simulink model "plane_stablizer_1"  (R2020b)
settings: Solver=VariableStepAuto  StartTime=0.0  StopTime=10.0  RelTol=1e-3
undefined symbols (not defined in the file): DiscIntNeverNeededParam
libraries: arduinolib x3, svdutilitieslib x1, arduinosensorlib x1
settings Model: Creator=Chas  LastModifiedBy=Chas

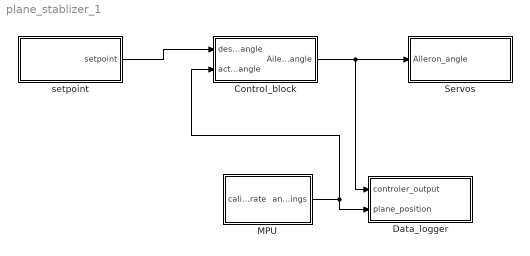
== system plane_stablizer_1 ==
  Control_block : Subsystem
  Data_logger : Subsystem
  MPU : Subsystem
  Servos : Subsystem
  setpoint : Subsystem
  wires:
  setpoint/1(setpoint) -> Control_block/1(desired_plane_angle)
  Control_block/1(Aileron_angle) -> Data_logger/1(controler_output), Servos/1(Aileron_angle)
  MPU/1(angle_of_wings) -> Control_block/2(actual_plan_angle), Data_logger/2(plane_position)

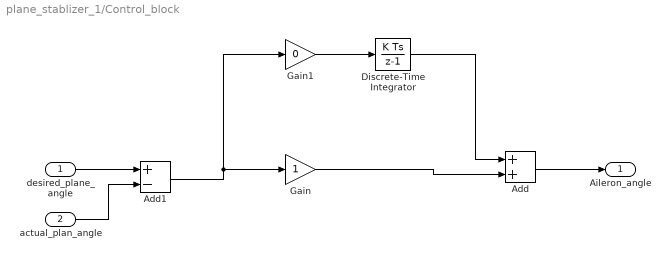
== system plane_stablizer_1/Control_block ==
  desired_plane_angle : Inport
  actual_plan_angle : Inport  Port=2
  Add : Sum
  Add1 : Sum  Inputs=+-
  Discrete-Time Integrator : DiscreteIntegrator  SampleTime=-1  ICPrevOutput=DiscIntNeverNeededParam  ICPrevScaledInput=DiscIntNeverNeededParam
  Gain : Gain
  Gain1 : Gain  Gain=0
  Aileron_angle : Outport
  wires:
  Gain1/1 -> Discrete-Time Integrator/1
  Discrete-Time Integrator/1 -> Add/1
  Gain/1 -> Add/2
  desired_plane_angle/1 -> Add1/1
  Add1/1 -> Gain1/1, Gain/1
  actual_plan_angle/1 -> Add1/2
  Add/1 -> Aileron_angle/1

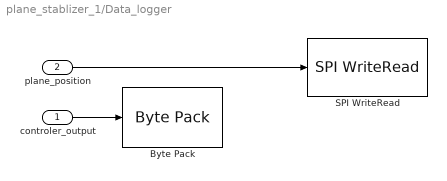
== system plane_stablizer_1/Data_logger ==
  controler_output : Inport
  plane_position : Inport  Port=2
  Byte Pack : svdutilitieslib/Byte Pack  maskPackedDataType=uint8  datatypes={'double'}  byteAlign=1  blockPlatform=arduinoert
      settings: SourceProductBaseCode=ANDROID,ARDUINO,ML_ARDUINO,ECCORTEXA,ECCORTEXR,SC_BEAGLEBONE_BLUE,EC_FREEDOM_BOARD,EC_FRDM_K64F,INTEL_BLOCKSET,JETSONCPU,MICROBIT,NUCLEO,NVIDIA,PX4AUTOPILOTS,RASPPIIO,STMICRODIS,TIC2000,XILINX_BLOCKSET
  SPI WriteRead : arduinolib/SPI WriteRead  slaveSelectPin_=10  blockPlatform=arduino
      settings: SourceProductBaseCode=ARDUINO
  wires:
  plane_position/1 -> SPI WriteRead/1
  controler_output/1 -> Byte Pack/1

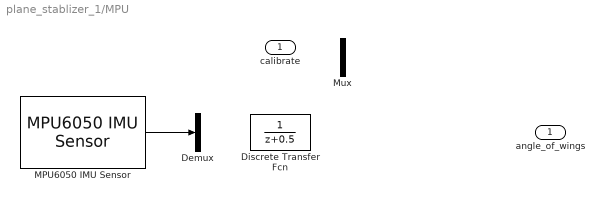
== system plane_stablizer_1/MPU ==
  calibrate : Inport
  Demux : Demux  Outputs=3
  Discrete Transfer Fcn : DiscreteTransferFcn
  MPU6050 IMU Sensor : arduinosensorlib/MPU6050 IMU Sensor  SlaveAddress=0x68  Accel=on  AngularRate=off  Temperature=off  Status=off  EulerAngles=off  Quat=off  AccelRange=2G  GyroRange=250 dps  DmpOdr=200 Hz  Dlpf=Accelerometer: 184Hz, Gyroscope: 188Hz  SampleTime=-1
      settings: SourceProductBaseCode=ARDUINO
  Mux : Mux  Inputs=2
  angle_of_wings : Outport
  wires:
  MPU6050 IMU Sensor/1 -> Demux/1

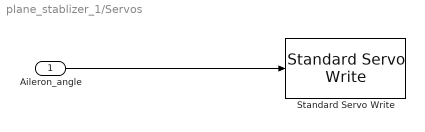
== system plane_stablizer_1/Servos ==
  Aileron_angle : Inport
  Standard Servo Write : arduinolib/Standard Servo Write  pinNumber=4  ServoIndex=0  blockPlatform=arduino
      settings: SourceProductName=Simulink Support Package for Arduino Hardware
  wires:
  Aileron_angle/1 -> Standard Servo Write/1

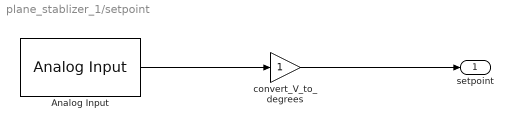
== system plane_stablizer_1/setpoint ==
  Analog Input : arduinolib/Analog Input  pinNumber=4  ReadResultsOnly=off  ConversionTriggerSource=Software  ExternalTriggerType=uint32( 0 )  OutputDataType=uint16  EnableConversionCompleteNotify=off  EnableOuputStatus=off  SampleTime=-1  blockPlatform=arduino
  convert_V_to_degrees : Gain
  setpoint : Outport
  wires:
  Analog Input/1 -> convert_V_to_degrees/1
  convert_V_to_degrees/1 -> setpoint/1
